simulink model "tanqueEsferico"  (R2014a)
settings: Solver=ode45  StartTime=0.0  StopTime=50  RelTol=1e-3
settings Model: Creator=gbtom  LastModifiedBy=gbtom

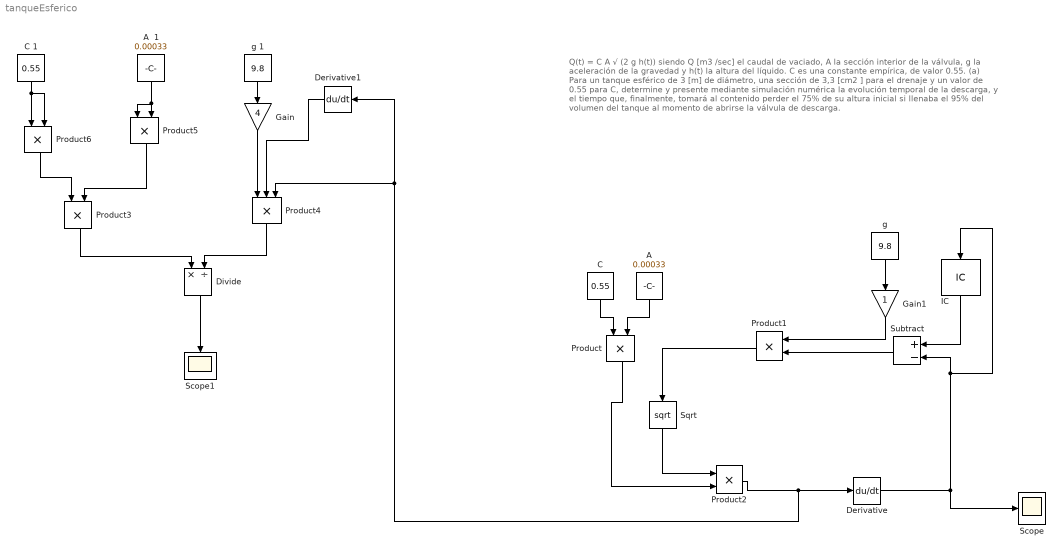
== system tanqueEsferico ==
  note: Q(t) = C A √ (2 g h(t))
      |
      | siendo Q [m3 /sec] el caudal de vaciado, A la sección interior de la válvula, g la aceleración de la gravedad y h(t) la altura del líquido.
      | C es una constante empírica, de valor 0.55. (a) Para un tanque esférico de 3 [m] de diámetro, una sección de 3,3 [cm2 ] para el drenaje
      | y un valor de 0.55 para C, determine y presente mediante simulación numérica la evolución temporal de la descarga, y el tiempo que,
      | finalmente, tomará al contenido perder el 75% de su altura inicial si llenaba el 95% del volumen del tanque al momento de abrirse
      | la válvula de descarga.
  "A  " : Constant  Value=0.00033
  A  1 : Constant  Value=0.00033
  "C " : Constant  Value=0.55
  C 1 : Constant  Value=0.55
  Derivative : Derivative
  Derivative1 : Derivative
  Divide : Product  Inputs=*/
  Gain : Gain  Gain=4
  Gain1 : Gain
  IC : InitialCondition  Value=14
  Product{,1..3,5..6} (6 alike) : Product
  Product4 : Product  Inputs=3
  Scope : Scope
      settings: ShowLegends=on  YMin=-15  YMax=155
  Scope1 : Scope
      settings: ShowLegends=on
  Sqrt : Sqrt  SaturateOnIntegerOverflow=on
  Subtract : Sum  Inputs=+-
  "g " : Constant  Value=9.8
  g 1 : Constant  Value=9.8
  wires:
  "C "/1 -> Product/1
  "A  "/1 -> Product/2
  Product1/1 -> Sqrt/1
  Sqrt/1 -> Product2/1
  Product/1 -> Product2/2
  A  1/1 -> Product5/1, Product5/2
  Product3/1 -> Divide/1
  Product5/1 -> Product3/2
  Product6/1 -> Product3/1
  C 1/1 -> Product6/2, Product6/1
  g 1/1 -> Gain/1
  Divide/1 -> Scope1/1
  Gain/1 -> Product4/1
  Product4/1 -> Divide/2
  "g "/1 -> Gain1/1
  Gain1/1 -> Product1/1
  Derivative1/1 -> Product4/2
  Product2/1 -> Derivative1/1, Product4/3, Derivative/1
  Subtract/1 -> Product1/2
  IC/1 -> Subtract/1
  Derivative/1 -> Scope/1, IC/1, Subtract/2
